simulink model "VOO"  (R2020a)
settings: Solver=FixedStepAuto  StartTime=0.0  StopTime=10.0  FixedStep=1e-3  RelTol=1e-3  EnableMultiTasking=on
undefined symbols (not defined in the file): D10, D12, D2, D3, D5, D7, D9, PTA1, PTA2, PTB9, PTC3, PTC4, PTD0, PTD3
libraries: frdmk64flib x7
settings Model: ExtModeTrigDuration=5  Creator=hinda  LastModifiedBy=hinda
settings OptimizationCC: EnhancedBackFolding=on  PassReuseOutputArgsAs=Individual arguments  ZeroExternalMemoryAtStartup=off  ZeroInternalMemoryAtStartup=off  MaxStackSize=64  OptimizeBlockOrder=speed  DifferentSizesBufferReuse=on  OptimizationCustomize=off  EfficientTunableParamExpr=on
settings DebuggingCC: ParameterTunabilityLossMsg=error
settings HardwareCC: ProdBitPerPointer=32  ProdBitPerSizeT=32  ProdBitPerPtrDiffT=32  ProdLargestAtomicInteger=Long  ProdLargestAtomicFloat=Double  ProdWordSize=32  ProdHWDeviceType=ARM Compatible->ARM Cortex
settings SFSimCC: MATLABDynamicMemAlloc=off
settings RTWCC: SystemTargetFile=ert.tlc  HardwareBoard=NXP FRDM-K64F  TemplateMakefile=ert_default_tmf  Toolchain=GNU Tools for ARM Embedded Processors
settings CodeAppCC: ForceParamTrailComments=on  IgnoreCustomStorageClasses=off  OperatorAnnotations=on  SimulinkDataObjDesc=on  SFDataObjDesc=on  InsertBlockDesc=on

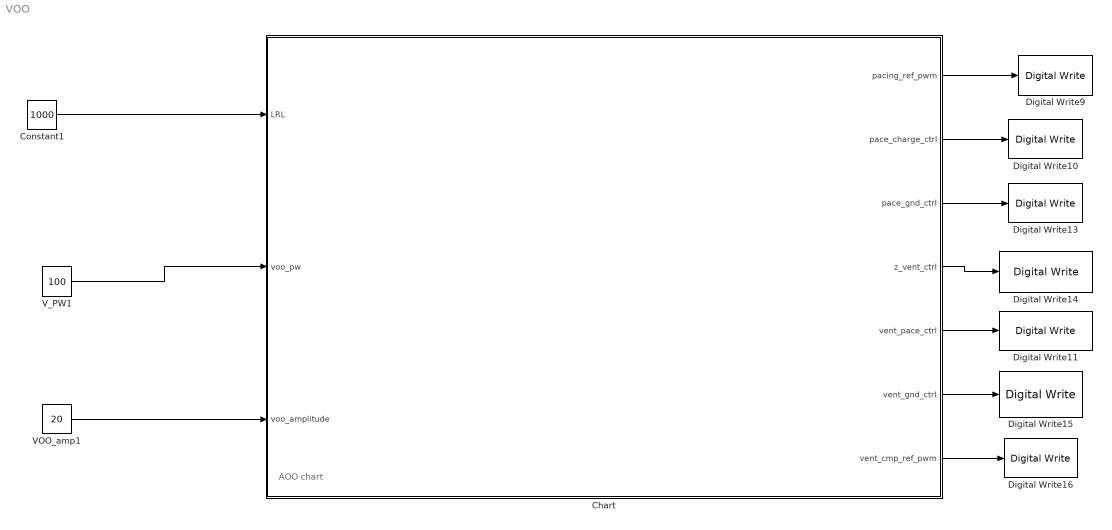
== system VOO ==
  note: AOO chart
  Chart : Stateflow chart  TreatAsAtomicUnit=on
  Constant1 : Constant  Value=1000
  Digital Write10 : frdmk64flib/Digital Write  Whichpin=PTB9 (D2)
  Digital Write11 : frdmk64flib/Digital Write  Whichpin=PTC4 (D9)
  Digital Write13 : frdmk64flib/Digital Write  Whichpin=PTD0 (D10)
  Digital Write14 : frdmk64flib/Digital Write  Whichpin=PTC3 (D7)
  Digital Write15 : frdmk64flib/Digital Write  Whichpin=PTD3 (D12)
  Digital Write16 : frdmk64flib/Digital Write  Whichpin=PTA1 (D3)
  Digital Write9 : frdmk64flib/Digital Write  Whichpin=PTA2 (D5)
  VOO_amp1 : Constant  Value=20
  V_PW1 : Constant  Value=100
  wires:
  Chart/7(vent_cmp_ref_pwm) -> Digital Write16/1
  Chart/5(vent_pace_ctrl) -> Digital Write11/1
  VOO_amp1/1 -> Chart/3(voo_amplitude)
  Chart/3(pace_gnd_ctrl) -> Digital Write13/1
  Constant1/1 -> Chart/1(LRL)
  Chart/4(z_vent_ctrl) -> Digital Write14/1
  Chart/2(pace_charge_ctrl) -> Digital Write10/1
  V_PW1/1 -> Chart/2(voo_pw)
  Chart/6(vent_gnd_ctrl) -> Digital Write15/1
  Chart/1(pacing_ref_pwm) -> Digital Write9/1

== stateflow chart VOO/Chart ==
  state charging
    entry:
    %charging C22
    %discharging C21
    vent_pace_ctrl = 0; %do not want c22 to discharge
    pacing_ref_pwm = voo_amplitude; %send in signal
    pace_charge_ctrl = 1;
    pace_gnd_ctrl = 0; %discharges C21
    vent_gnd_ctrl = 1; %1 when discharging through atrium
    vent_cmp_ref_pwm = 80; %send in threshold signal, if heart is less then we will send signal, idk
    %average threshold amplitude is 80
    z_vent_ctrl = 0; %connects impedance circuit to atrium ring electrode output is at z_signal pin
  state pacing
    entry:
    %charging C21
    %discharging C22
    vent_gnd_ctrl = 0;
    vent_pace_ctrl = 1;
    z_vent_ctrl = 0;
    pace_charge_ctrl = 0;
    pace_gnd_ctrl = 1;
    vent_gnd_ctrl = 0;
    pacing_ref_pwm = voo_amplitude;
  (default) -> charging
  charging -> pacing : [after(voo_pw, msec)]
  pacing -> charging : [after(LRL - voo_pw, msec)]
  data: LRL input; pacing_ref_pwm output; pace_charge_ctrl output; pace_gnd_ctrl output; z_vent_ctrl output; vent_pace_ctrl output; vent_gnd_ctrl output; vent_cmp_ref_pwm output; voo_pw input; voo_amplitude input
